simulink model "EHB_MOTOR"  (R2023b)
settings: Solver=FixedStepDiscrete  StartTime=0.0  StopTime=inf  FixedStep=0.0001  RelTol=1e-3  EnableMultiTasking=on
undefined symbols (not defined in the file): CAN_EHB_VCU0x125, CAN_EHB_VCU0x126, CAN_id0x120_Data, Cos_Table, Cos_Table1, EHB_DTC_status, R, Sin_BreakPoint, Sin_BreakPoint1, Sin_Table, Sin_Table1, T
libraries: simulink x30
(part 2 of 9)

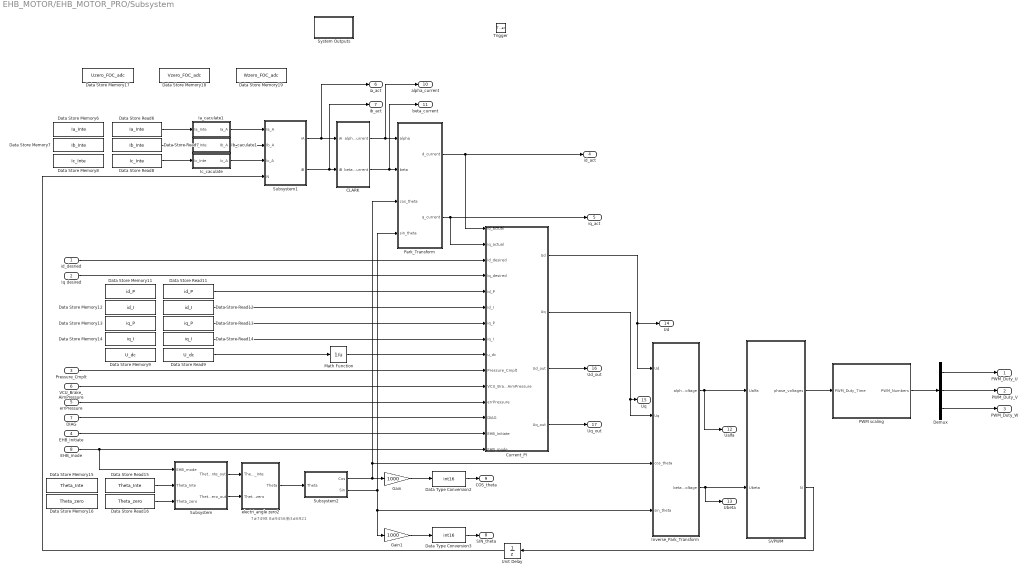
== system EHB_MOTOR/EHB_MOTOR_PRO/Subsystem ==
  note: 7#7498
      | 8#9456
      | 新3#6921
  id_desried : Inport
  Iq desired : Inport  Port=2  OutDataTypeStr=single
  Pressure_Cmplt : Inport  Port=3
  EHB_Initiate : Inport  Port=4
  errPressure : Inport  Port=5
  VCU_Brake_AimPressure : Inport  Port=6
  DIAG : Inport  Port=7
  EHB_mode : Inport  Port=8
  Trigger : TriggerPort  TriggerType=function-call  VariantControl=Variant  PortDimensions=1
  CLARK : Subsystem
  Current_PI : Subsystem
  Data Store Memory11 : DataStoreMemory  DataStoreName=id_P  ReadBeforeWriteMsg=warning  WriteAfterWriteMsg=warning  WriteAfterReadMsg=warning  ShowAdditionalParam=off  OutDataTypeStr=single
  Data Store Memory12 : DataStoreMemory  DataStoreName=id_I  ReadBeforeWriteMsg=warning  WriteAfterWriteMsg=warning  WriteAfterReadMsg=warning  ShowAdditionalParam=off  OutDataTypeStr=single
  Data Store Memory13 : DataStoreMemory  DataStoreName=iq_P  ReadBeforeWriteMsg=warning  WriteAfterWriteMsg=warning  WriteAfterReadMsg=warning  ShowAdditionalParam=off  OutDataTypeStr=single
  Data Store Memory14 : DataStoreMemory  DataStoreName=iq_I  ReadBeforeWriteMsg=warning  WriteAfterWriteMsg=warning  WriteAfterReadMsg=warning  ShowAdditionalParam=off  OutDataTypeStr=single
  Data Store Memory15 : DataStoreMemory  DataStoreName=Theta_Inte  ReadBeforeWriteMsg=warning  WriteAfterWriteMsg=warning  WriteAfterReadMsg=warning  ShowAdditionalParam=off  OutDataTypeStr=uint16
  Data Store Memory16 : DataStoreMemory  DataStoreName=Theta_zero  ReadBeforeWriteMsg=warning  WriteAfterWriteMsg=warning  WriteAfterReadMsg=warning  ShowAdditionalParam=off  OutDataTypeStr=uint16
  Data Store Memory17 : DataStoreMemory  DataStoreName=Uzero_FOC_adc  ReadBeforeWriteMsg=warning  WriteAfterWriteMsg=warning  WriteAfterReadMsg=warning  ShowAdditionalParam=off  OutDataTypeStr=uint16
  Data Store Memory18 : DataStoreMemory  DataStoreName=Vzero_FOC_adc  ReadBeforeWriteMsg=warning  WriteAfterWriteMsg=warning  WriteAfterReadMsg=warning  ShowAdditionalParam=off  OutDataTypeStr=uint16
  Data Store Memory19 : DataStoreMemory  DataStoreName=Wzero_FOC_adc  ReadBeforeWriteMsg=warning  WriteAfterWriteMsg=warning  WriteAfterReadMsg=warning  ShowAdditionalParam=off  OutDataTypeStr=uint16
  Data Store Memory6 : DataStoreMemory  DataStoreName=Ia_Inte  ReadBeforeWriteMsg=warning  WriteAfterWriteMsg=warning  WriteAfterReadMsg=warning  ShowAdditionalParam=off  OutDataTypeStr=uint16
  Data Store Memory7 : DataStoreMemory  DataStoreName=Ib_Inte  ReadBeforeWriteMsg=warning  WriteAfterWriteMsg=warning  WriteAfterReadMsg=warning  ShowAdditionalParam=off  OutDataTypeStr=uint16
  Data Store Memory8 : DataStoreMemory  DataStoreName=Ic_Inte  ReadBeforeWriteMsg=warning  WriteAfterWriteMsg=warning  WriteAfterReadMsg=warning  ShowAdditionalParam=off  OutDataTypeStr=uint16
  Data Store Memory9 : DataStoreMemory  DataStoreName=U_dc  ReadBeforeWriteMsg=warning  WriteAfterWriteMsg=warning  WriteAfterReadMsg=warning  ShowAdditionalParam=off  OutDataTypeStr=single
  Data Store Read11 : DataStoreRead  DataStoreName=id_P  DataStoreElements=id_P  IndexOptions=Index vector (dialog)  Indices=1  OutputSizes=1
  Data Store Read12 : DataStoreRead  DataStoreName=id_I  DataStoreElements=id_I  IndexOptions=Index vector (dialog)  Indices=1  OutputSizes=1
  Data Store Read13 : DataStoreRead  DataStoreName=iq_P  DataStoreElements=iq_P  IndexOptions=Index vector (dialog)  Indices=1  OutputSizes=1
  Data Store Read14 : DataStoreRead  DataStoreName=iq_I  DataStoreElements=iq_I  IndexOptions=Index vector (dialog)  Indices=1  OutputSizes=1
  Data Store Read15 : DataStoreRead  DataStoreName=Theta_Inte  DataStoreElements=Theta_Inte  IndexOptions=Index vector (dialog)  Indices=1  OutputSizes=1
  Data Store Read16 : DataStoreRead  DataStoreName=Theta_zero  DataStoreElements=Theta_zero  IndexOptions=Index vector (dialog)  Indices=1  OutputSizes=1
  Data Store Read6 : DataStoreRead  DataStoreName=Ia_Inte  DataStoreElements=Ia_Inte  IndexOptions=Index vector (dialog)  Indices=1  OutputSizes=1
  Data Store Read7 : DataStoreRead  DataStoreName=Ib_Inte  DataStoreElements=Ib_Inte  IndexOptions=Index vector (dialog)  Indices=1  OutputSizes=1
  Data Store Read8 : DataStoreRead  DataStoreName=Ic_Inte  DataStoreElements=Ic_Inte  IndexOptions=Index vector (dialog)  Indices=1  OutputSizes=1
  Data Store Read9 : DataStoreRead  DataStoreName=U_dc  DataStoreElements=U_dc  IndexOptions=Index vector (dialog)  Indices=1  OutputSizes=1
  Data Type Conversion2 : DataTypeConversion  OutDataTypeStr=int16  SaturateOnIntegerOverflow=off  RndMeth=Floor
  Data Type Conversion3 : DataTypeConversion  OutDataTypeStr=int16  SaturateOnIntegerOverflow=off  RndMeth=Floor
  Demux : Demux  Outputs=3
  Gain : Gain  Gain=1000
  Gain1 : Gain  Gain=1000
  Ia_caculate1 : Subsystem
  Ib_caculate1 : Subsystem
  Ic_caculate : Subsystem
  Inverse_Park_Transform : Subsystem
  Math Function : Math  Operator=reciprocal  SignedPower=on  OutDataTypeStr=single
  PWM scaling : Subsystem
  Park_Transform : Subsystem
  SVPWM : Subsystem
  Subsystem : Subsystem
  Subsystem1 : Subsystem
  Subsystem2 : Subsystem
  System Outputs : Subsystem  mask(System Outputs){ShowInLibBrowser=0}
      mask prompts: ShowInLibBrowser "Simulink:masks:CustCodeMaskParam1_MP"
      settings: CopyFcn=cccopyfcn(gcb)  OpenFcn=ccopenfcn('System Outputs Function')
      mask Help: eval('feval(''rtwprivate'',''rtwhelpview'',''rtw_sys_outputs_block'')');
      mask Display: disp('System\nOutputs');
  Unit Delay : UnitDelay  SampleTime=-1  HasFrameUpgradeWarning=on
  electri_angle zero2 : Subsystem
  PWM_Duty_U : Outport  VectorParamsAs1DForOutWhenUnconnected=off
  PWM_Duty_V : Outport  Port=2  VectorParamsAs1DForOutWhenUnconnected=off
  PWM_Duty_W : Outport  Port=3  VectorParamsAs1DForOutWhenUnconnected=off
  id_act : Outport  Port=4  VectorParamsAs1DForOutWhenUnconnected=off
  iq_act : Outport  Port=5  VectorParamsAs1DForOutWhenUnconnected=off
  ia_act : Outport  Port=6  OutDataTypeStr=single  VectorParamsAs1DForOutWhenUnconnected=off
  ib_act : Outport  Port=7  OutDataTypeStr=single  VectorParamsAs1DForOutWhenUnconnected=off
  SIN_theta : Outport  Port=8  VectorParamsAs1DForOutWhenUnconnected=off
  COS_theta : Outport  Port=9  VectorParamsAs1DForOutWhenUnconnected=off
  alpha_current : Outport  Port=10  OutDataTypeStr=single  VectorParamsAs1DForOutWhenUnconnected=off
  beta_current : Outport  Port=11  OutDataTypeStr=single  VectorParamsAs1DForOutWhenUnconnected=off
  Ualfa : Outport  Port=12  VectorParamsAs1DForOutWhenUnconnected=off
  Ubeta : Outport  Port=13  VectorParamsAs1DForOutWhenUnconnected=off
  Ud : Outport  Port=14  VectorParamsAs1DForOutWhenUnconnected=off
  Uq : Outport  Port=15  VectorParamsAs1DForOutWhenUnconnected=off
  Ud_out : Outport  Port=16  OutDataTypeStr=single  VectorParamsAs1DForOutWhenUnconnected=off
  Uq_out : Outport  Port=17  OutDataTypeStr=single  VectorParamsAs1DForOutWhenUnconnected=off
  wires:
  Inverse_Park_Transform/2(beta_voltage) -> Ubeta/1, SVPWM/2(Ubeta)
  Iq desired/1 -> Current_PI/4(Iq_desired)
  Data Store Read13/1 -> Current_PI/7(iq_P)
  CLARK/1(alpha_current) -> alpha_current/1, Park_Transform/1(alpha)
  Demux/1 -> PWM_Duty_U/1
  CLARK/2(beta_current) -> beta_current/1, Park_Transform/2(beta)
  Data Store Read12/1 -> Current_PI/6(id_I)
  Data Store Read14/1 -> Current_PI/8(iq_I)
  Park_Transform/2(q_current) -> Current_PI/2(iq_actual), iq_act/1
  Current_PI/2(Uq) -> Inverse_Park_Transform/2(Uq), Uq/1
  Data Store Read11/1 -> Current_PI/5(id_P)
  Math Function/1 -> Current_PI/9(u_dc)
  Gain1/1 -> Data Type Conversion3/1
  Gain/1 -> Data Type Conversion2/1
  Inverse_Park_Transform/1(alpha_voltage) -> Ualfa/1, SVPWM/1(Ualfa)
  Current_PI/1(Ud) -> Inverse_Park_Transform/1(Ud), Ud/1
  Data Type Conversion3/1 -> SIN_theta/1
  Subsystem1/1(iA) -> ia_act/1, CLARK/1(iA)
  PWM scaling/1(PWM_Numbers) -> Demux/1
  Park_Transform/1(d_current) -> Current_PI/1(id_actual), id_act/1
  Subsystem1/2(iB) -> ib_act/1, CLARK/2(iB)
  Demux/3 -> PWM_Duty_W/1
  Data Store Read7/1 -> Ib_caculate1/1(Ib_Inte)
  Data Store Read6/1 -> Ia_caculate1/1(Ia_Inte)
  Data Store Read9/1 -> Math Function/1
  Demux/2 -> PWM_Duty_V/1
  Data Type Conversion2/1 -> COS_theta/1
  id_desried/1 -> Current_PI/3(id_desired)
  SVPWM/1(phase_voltages) -> PWM scaling/1(PWM_Duty_Time)
  Pressure_Cmplt/1 -> Current_PI/10(Pressure_Cmplt)
  VCU_Brake_AimPressure/1 -> Current_PI/11(VCU_Brake_AimPressure)
  Ib_caculate1/1(Ib_A) -> Subsystem1/2(Ib_A)
  Ia_caculate1/1(Ia_A) -> Subsystem1/1(Ia_A)
  Ic_caculate/1(Ic_A) -> Subsystem1/3(Ic_A)
  Data Store Read8/1 -> Ic_caculate/1(Ic_Inte)
  SVPWM/2(N) -> Unit Delay/1
  Unit Delay/1 -> Subsystem1/4(N)
  Subsystem2/1(Cos) -> Park_Transform/3(cos_theta), Inverse_Park_Transform/3(cos_theta), Gain/1
  Subsystem2/2(Sin) -> Gain1/1, Inverse_Park_Transform/4(sin_theta), Park_Transform/4(sin_theta)
  electri_angle zero2/1(Theta) -> Subsystem2/1(Theta)
  errPressure/1 -> Current_PI/12(errPressure)
  DIAG/1 -> Current_PI/13(DIAG)
  EHB_Initiate/1 -> Current_PI/14(EHB_Initiate)
  EHB_mode/1 -> Subsystem/1(EHB_mode), Current_PI/15(EHB_mode)
  Data Store Read15/1 -> Subsystem/2(Theta_Inte)
  Data Store Read16/1 -> Subsystem/3(Theta_zero)
  Subsystem/1(Theta_Inte_out) -> electri_angle zero2/1(Theta_Inte)
  Subsystem/2(Theta_zero_out) -> electri_angle zero2/2(Theta_zero)
  Current_PI/4(Uq_out) -> Uq_out/1
  Current_PI/3(Ud_out) -> Ud_out/1

== system EHB_MOTOR/EPB_CTRL/EPB_CTRL ==
  EPB_CMD : Inport
  EPB_DiagBUS : Inport  Port=2
  EPB_INPUTBUS : Inport  Port=3
  Trigger : TriggerPort  TriggerType=function-call  VariantControl=Variant  PortDimensions=1
  Bus Selector : BusSelector  OutputSignals=EPB1_Current_filtered,EPB2_Current_filtered
  Chart : Stateflow chart  TreatAsAtomicUnit=on
  Constant : Constant  Value=0  OutDataTypeStr=uint8
  Data Store Memory1 : DataStoreMemory  DataStoreName=EPB_tiRelease_C  ReadBeforeWriteMsg=warning  WriteAfterWriteMsg=warning  WriteAfterReadMsg=warning  ShowAdditionalParam=off  OutDataTypeStr=uint16
  Data Store Memory2 : DataStoreMemory  DataStoreName=EPB_tiClamp_C  ReadBeforeWriteMsg=warning  WriteAfterWriteMsg=warning  WriteAfterReadMsg=warning  ShowAdditionalParam=off  OutDataTypeStr=uint16
  Data Store Memory3 : DataStoreMemory  DataStoreName=EPB1_iAct_C  ReadBeforeWriteMsg=warning  WriteAfterWriteMsg=warning  WriteAfterReadMsg=warning  ShowAdditionalParam=off  OutDataTypeStr=single
  Data Store Memory4 : DataStoreMemory  DataStoreName=EPB2_iAct_C  ReadBeforeWriteMsg=warning  WriteAfterWriteMsg=warning  WriteAfterReadMsg=warning  ShowAdditionalParam=off  OutDataTypeStr=single
  Data Store Read : DataStoreRead  DataStoreName=EPB_tiClamp_C  DataStoreElements=EPB_tiClamp_C  IndexOptions=Index vector (dialog)  Indices=1  OutputSizes=1
  Data Store Read1 : DataStoreRead  DataStoreName=EPB_tiRelease_C  DataStoreElements=EPB_tiRelease_C  IndexOptions=Index vector (dialog)  Indices=1  OutputSizes=1
  Data Store Read2 : DataStoreRead  DataStoreName=EPB1_iAct_C  DataStoreElements=EPB1_iAct_C  IndexOptions=Index vector (dialog)  Indices=1  OutputSizes=1
  Data Store Read3 : DataStoreRead  DataStoreName=EPB2_iAct_C  DataStoreElements=EPB2_iAct_C  IndexOptions=Index vector (dialog)  Indices=1  OutputSizes=1
  Fault_Handle : Subsystem
  Switch : Switch  Criteria=u2 ~= 0  SaturateOnIntegerOverflow=off  InputSameDT=off
  EPB_PWMout : Outport  VectorParamsAs1DForOutWhenUnconnected=off
  EPB_state : Outport  Port=2  VectorParamsAs1DForOutWhenUnconnected=off
  Clamp_ok : Outport  Port=3  VectorParamsAs1DForOutWhenUnconnected=off
  Release_ok : Outport  Port=4  VectorParamsAs1DForOutWhenUnconnected=off
  wires:
  EPB_INPUTBUS/1 -> Bus Selector/1
  EPB_CMD/1 -> Chart/1(EPB_Ctrl_Req)
  Bus Selector/1 -> Chart/2(EPB1_iAct)  "<EPB1_Current_filtered>"
  Bus Selector/2 -> Chart/3(EPB2_iAct)  "<EPB2_Current_filtered>"
  Data Store Read/1 -> Chart/4(EPB_tiClamp_C)
  Data Store Read1/1 -> Chart/5(EPB_tiRelease_C)
  Data Store Read2/1 -> Chart/6(EPB1_iAct_C)
  Data Store Read3/1 -> Chart/7(EPB2_iAct_C)
  Chart/1(EPB_PWMout) -> Switch/3
  Chart/2(EPB_dir_state) -> EPB_state/1
  Chart/3(Clamp_ok) -> Clamp_ok/1
  Chart/4(Release_ok) -> Release_ok/1
  EPB_DiagBUS/1 -> Fault_Handle/1(In1)
  Fault_Handle/1(Out1) -> Switch/2
  Constant/1 -> Switch/1
  Switch/1 -> EPB_PWMout/1

== system EHB_MOTOR/EPB_CTRL/EPB_Diag ==
  In1 : Inport
  Trigger : TriggerPort  TriggerType=function-call  VariantControl=Variant  PortDimensions=1
  Bus Creator : BusCreator  Inputs=4
  Bus Selector13 : BusSelector  OutputSignals=EPB1_Current_filtered,EPB2_Current_filtered
  Bus Selector15 : BusSelector  OutputSignals=EPB1_Temp
  Bus Selector5 : BusSelector  OutputSignals=EPB_vBAT_filtered
  EPBCurrentDiag : Subsystem
  EPBOverheatDiag : Subsystem
  EPB_vBATDiag : Subsystem
  EPB_DiagBUS : Outport  VectorParamsAs1DForOutWhenUnconnected=off
  wires:
  Bus Selector5/1 -> EPB_vBATDiag/1(EPBVoltage)  "<EPB_vBAT_filtered>"
  Bus Selector15/1 -> EPBOverheatDiag/1(EPBTemp)  "<EPB1_Temp>"
  Bus Selector13/2 -> EPBCurrentDiag/2(EPB2Current)  "<EPB2_Current_filtered>"
  Bus Selector13/1 -> EPBCurrentDiag/1(EPB1Current)  "<EPB1_Current_filtered>"
  In1/1 -> Bus Selector13/1, Bus Selector15/1, Bus Selector5/1
  EPB_vBATDiag/1(EPBVoltageLow) -> Bus Creator/1  "EPBVoltageLow"
  EPB_vBATDiag/2(EPBVoltageHigh) -> Bus Creator/2  "EPBVoltageHigh"
  EPBOverheatDiag/1(EPBOverheat) -> Bus Creator/3  "EPBOverheat"
  EPBCurrentDiag/1(EPBCurrentOverride) -> Bus Creator/4  "EPBCurrentOverride"
  Bus Creator/1 -> EPB_DiagBUS/1

== system EHB_MOTOR/EPB_CTRL/Subsystem1 ==
  Trigger : TriggerPort  TriggerType=function-call  VariantControl=Variant  PortDimensions=1
  Bus Creator : BusCreator  Inputs=11
  Data Store Memory11 : DataStoreMemory  DataStoreName=EPB_vBAT_AD  ReadBeforeWriteMsg=warning  WriteAfterWriteMsg=warning  WriteAfterReadMsg=warning  ShowAdditionalParam=off  OutDataTypeStr=uint16
  Data Store Memory12 : DataStoreMemory  DataStoreName=EPB1_Temp_AD  ReadBeforeWriteMsg=warning  WriteAfterWriteMsg=warning  WriteAfterReadMsg=warning  ShowAdditionalParam=off  OutDataTypeStr=uint16
  Data Store Memory13 : DataStoreMemory  DataStoreName=EPB_APBSwitch2_AD  ReadBeforeWriteMsg=warning  WriteAfterWriteMsg=warning  WriteAfterReadMsg=warning  ShowAdditionalParam=off  OutDataTypeStr=uint16
  Data Store Memory14 : DataStoreMemory  DataStoreName=EPB_7181PreDriver1_AD  ReadBeforeWriteMsg=warning  WriteAfterWriteMsg=warning  WriteAfterReadMsg=warning  ShowAdditionalParam=off  OutDataTypeStr=uint16
  Data Store Memory15 : DataStoreMemory  DataStoreName=EPB2_Temp_AD  ReadBeforeWriteMsg=warning  WriteAfterWriteMsg=warning  WriteAfterReadMsg=warning  ShowAdditionalParam=off  OutDataTypeStr=uint16
  Data Store Memory17 : DataStoreMemory  DataStoreName=EPB_APBSwitch3_AD  ReadBeforeWriteMsg=warning  WriteAfterWriteMsg=warning  WriteAfterReadMsg=warning  ShowAdditionalParam=off  OutDataTypeStr=uint16
  Data Store Memory18 : DataStoreMemory  DataStoreName=EPB_APBSwitch4_AD  ReadBeforeWriteMsg=warning  WriteAfterWriteMsg=warning  WriteAfterReadMsg=warning  ShowAdditionalParam=off  OutDataTypeStr=uint16
  Data Store Memory19 : DataStoreMemory  DataStoreName=EPB2_Current_AD  ReadBeforeWriteMsg=warning  WriteAfterWriteMsg=warning  WriteAfterReadMsg=warning  ShowAdditionalParam=off  OutDataTypeStr=uint16
  Data Store Memory20 : DataStoreMemory  DataStoreName=EPB_APBSwitch1_AD  ReadBeforeWriteMsg=warning  WriteAfterWriteMsg=warning  WriteAfterReadMsg=warning  ShowAdditionalParam=off  OutDataTypeStr=uint16
  Data Store Memory21 : DataStoreMemory  DataStoreName=EPB1_Current_AD  ReadBeforeWriteMsg=warning  WriteAfterWriteMsg=warning  WriteAfterReadMsg=warning  ShowAdditionalParam=off  OutDataTypeStr=uint16
  Data Store Memory22 : DataStoreMemory  DataStoreName=EPB_7181PreDriver2_AD  ReadBeforeWriteMsg=warning  WriteAfterWriteMsg=warning  WriteAfterReadMsg=warning  ShowAdditionalParam=off  OutDataTypeStr=uint16
  Data Store Read11 : DataStoreRead  DataStoreName=EPB_vBAT_AD  DataStoreElements=EPB_vBAT_AD  IndexOptions=Index vector (dialog)  Indices=1  OutputSizes=1
  Data Store Read12 : DataStoreRead  DataStoreName=EPB1_Temp_AD  DataStoreElements=EPB1_Temp_AD  IndexOptions=Index vector (dialog)  Indices=1  OutputSizes=1
  Data Store Read13 : DataStoreRead  DataStoreName=EPB_APBSwitch2_AD  DataStoreElements=EPB_APBSwitch2_AD  IndexOptions=Index vector (dialog)  Indices=1  OutputSizes=1
  Data Store Read14 : DataStoreRead  DataStoreName=EPB_7181PreDriver1_AD  DataStoreElements=EPB_7181PreDriver1_AD  IndexOptions=Index vector (dialog)  Indices=1  OutputSizes=1
  Data Store Read15 : DataStoreRead  DataStoreName=EPB2_Temp_AD  DataStoreElements=EPB2_Temp_AD  IndexOptions=Index vector (dialog)  Indices=1  OutputSizes=1
  Data Store Read17 : DataStoreRead  DataStoreName=EPB_APBSwitch3_AD  DataStoreElements=EPB_APBSwitch3_AD  IndexOptions=Index vector (dialog)  Indices=1  OutputSizes=1
  Data Store Read18 : DataStoreRead  DataStoreName=EPB_APBSwitch4_AD  DataStoreElements=EPB_APBSwitch4_AD  IndexOptions=Index vector (dialog)  Indices=1  OutputSizes=1
  Data Store Read19 : DataStoreRead  DataStoreName=EPB2_Current_AD  DataStoreElements=EPB2_Current_AD  IndexOptions=Index vector (dialog)  Indices=1  OutputSizes=1
  Data Store Read20 : DataStoreRead  DataStoreName=EPB_APBSwitch1_AD  DataStoreElements=EPB_APBSwitch1_AD  IndexOptions=Index vector (dialog)  Indices=1  OutputSizes=1
  Data Store Read21 : DataStoreRead  DataStoreName=EPB1_Current_AD  DataStoreElements=EPB1_Current_AD  IndexOptions=Index vector (dialog)  Indices=1  OutputSizes=1
  Data Store Read22 : DataStoreRead  DataStoreName=EPB_7181PreDriver2_AD  DataStoreElements=EPB_7181PreDriver2_AD  IndexOptions=Index vector (dialog)  Indices=1  OutputSizes=1
  EPB_interface : Subsystem
  EPB_INPUTBUS : Outport  VectorParamsAs1DForOutWhenUnconnected=off
  wires:
  Data Store Read21/1 -> EPB_interface/2(EPB1_Current_AD)
  Data Store Read17/1 -> EPB_interface/6(EPB_APBSwitch3_AD)
  Data Store Read14/1 -> EPB_interface/11(EPB_7181PreDriver1_AD)
  Data Store Read13/1 -> EPB_interface/10(EPB_7181PreDriver2_AD)
  EPB_interface/9(EPB_APBSwitch2_filtered) -> Bus Creator/9  "EPB_7181PreDriver2_filtered"
  Data Store Read19/1 -> EPB_interface/3(EPB2_Current_AD)
  Data Store Read12/1 -> EPB_interface/4(EPB1_Temp_AD)
  Data Store Read22/1 -> EPB_interface/9(EPB_APBSwitch2_AD)
  Data Store Read15/1 -> EPB_interface/5(EPB2_Temp_AD)
  Data Store Read20/1 -> EPB_interface/8(EPB_APBSwitch1_AD)
  EPB_interface/7(EPB_APBSwitch4_filtered) -> Bus Creator/7  "EPB_APBSwitch4_filtered"
  EPB_interface/11(EPB_7181PreDriver1_filtered) -> Bus Creator/11  "EPB_7181PreDriver1_filtered"
  EPB_interface/4(EPB1_Temp) -> Bus Creator/4  "EPB1_Temp"
  EPB_interface/3(EPB2_Current_filtered) -> Bus Creator/3  "EPB2_Current_filtered"
  Data Store Read11/1 -> EPB_interface/1(EPB_vBAT_AD)
  EPB_interface/2(EPB1_Current_filtered) -> Bus Creator/2  "EPB1_Current_filtered"
  Data Store Read18/1 -> EPB_interface/7(EPB_APBSwitch4_AD)
  EPB_interface/6(EPB_APBSwitch3_filtered) -> Bus Creator/6  "EPB_APBSwitch3_filtered"
  EPB_interface/5(EPB2_Temp) -> Bus Creator/5  "EPB2_Temp"
  EPB_interface/1(EPB_vBAT_filtered) -> Bus Creator/1  "EPB_vBAT_filtered"
  EPB_interface/10(EPB_7181PreDriver2_filtered) -> Bus Creator/10  "EPB_APBSwitch2_filtered"
  EPB_interface/8(EPB_APBSwitch1_filtered) -> Bus Creator/8  "EPB_APBSwitch1_filtered"
  Bus Creator/1 -> EPB_INPUTBUS/1

== system EHB_MOTOR/EHB_MOTOR_PRO/DIAG/5vDiag ==
  note: 20ms
  note: 5v输出异常
  5vVoltage : Inport
  Chart : Stateflow chart  TreatAsAtomicUnit=on
  Subsystem : Subsystem
  5vErr : Outport  VectorParamsAs1DForOutWhenUnconnected=off
  wires:
  5vVoltage/1 -> Subsystem/1(In1)
  Subsystem/1(Out1) -> 5vErr/1
  Chart/1(task_20ms()) -> Subsystem/Trigger

== system EHB_MOTOR/EHB_MOTOR_PRO/DIAG/AngleSensorDiag ==
  note: 角度传感器缺少标定
  note: 角度传感器没有信号
  note: 200ms
  note: 角度传感器信号超限故障
  note: 200ms
  note: 200ms
  AngleSensorSignal : Inport
  AngleSensorCalFlag : Inport  Port=2
  Chart : Stateflow chart  TreatAsAtomicUnit=on
  Chart1 : Stateflow chart  TreatAsAtomicUnit=on
  Chart2 : Stateflow chart  TreatAsAtomicUnit=on
  Subsystem : Subsystem
  Subsystem1 : Subsystem
  Subsystem2 : Subsystem
  AngleSensorSignalOverride : Outport  VectorParamsAs1DForOutWhenUnconnected=off
  AngleSensorSignalLost : Outport  Port=2  VectorParamsAs1DForOutWhenUnconnected=off
  AngleSensorNoCal : Outport  Port=3  VectorParamsAs1DForOutWhenUnconnected=off
  wires:
  Subsystem/1(Out1) -> AngleSensorSignalOverride/1
  Chart/1(task_200ms()) -> Subsystem/Trigger
  Chart1/1(task_200ms()) -> Subsystem1/Trigger
  Subsystem1/1(Out1) -> AngleSensorSignalLost/1
  AngleSensorSignal/1 -> Subsystem1/1(In1), Subsystem/1(In1)
  Subsystem2/1(Out1) -> AngleSensorNoCal/1
  Chart2/1(task_200ms()) -> Subsystem2/Trigger
  AngleSensorCalFlag/1 -> Subsystem2/1(In1)

== system EHB_MOTOR/EHB_MOTOR_PRO/DIAG/BusOffDiag ==
  note: 控制器内部故障
  In1 : Inport
  Ground : Ground
  Terminator : Terminator
  BusOffErr : Outport  VectorParamsAs1DForOutWhenUnconnected=off
  wires:
  In1/1 -> Terminator/1
  Ground/1 -> BusOffErr/1

== system EHB_MOTOR/EHB_MOTOR_PRO/DIAG/CANCommDiag ==
  note: CAN收发模块故障
  In1 : Inport
  Ground : Ground
  Terminator : Terminator
  CANCommErr : Outport  VectorParamsAs1DForOutWhenUnconnected=off
  wires:
  In1/1 -> Terminator/1
  Ground/1 -> CANCommErr/1

== system EHB_MOTOR/EHB_MOTOR_PRO/DIAG/CANDataLostDiag ==
  note: CAN丢失数据
  In1 : Inport
  Ground : Ground
  Terminator : Terminator
  CANDataLostErr : Outport  VectorParamsAs1DForOutWhenUnconnected=off
  wires:
  In1/1 -> Terminator/1
  Ground/1 -> CANDataLostErr/1

== system EHB_MOTOR/EHB_MOTOR_PRO/DIAG/Chip7189Diag ==
  note: 7189芯片故障
  note: 20ms
  Chart : Stateflow chart  TreatAsAtomicUnit=on
  Data Store Memory1 : DataStoreMemory  DataStoreName=Chip7189ErrFlag  ReadBeforeWriteMsg=warning  WriteAfterWriteMsg=warning  WriteAfterReadMsg=warning  ShowAdditionalParam=off  OutDataTypeStr=uint8
  Data Store Read2 : DataStoreRead  DataStoreName=Chip7189ErrFlag  DataStoreElements=Chip7189ErrFlag  IndexOptions=Index vector (dialog)  Indices=1  OutputSizes=1
  Subsystem : Subsystem
  Chip7189_err : Outport  VectorParamsAs1DForOutWhenUnconnected=off
  wires:
  Chart/1(task_20ms()) -> Subsystem/Trigger
  Subsystem/1(Out1) -> Chip7189_err/1
  Data Store Read2/1 -> Subsystem/1(In1)

== system EHB_MOTOR/EHB_MOTOR_PRO/DIAG/CurrentSensorDiag ==
  note: 200ms
  note: U相电流传感器故障
  note: 200ms
  note: V相电流传感器故障
  note: 200ms
  note: W相电流传感器故障
  CurrentSensorU : Inport
  CurrentSensorV : Inport  Port=2
  CurrentSensorW : Inport  Port=3
  Chart : Stateflow chart  TreatAsAtomicUnit=on
  Chart1 : Stateflow chart  TreatAsAtomicUnit=on
  Chart2 : Stateflow chart  TreatAsAtomicUnit=on
  Subsystem : Subsystem
  Subsystem1 : Subsystem
  Subsystem2 : Subsystem
  CurrentSensorUOverride : Outport  VectorParamsAs1DForOutWhenUnconnected=off
  CurrentSensorVOverride : Outport  Port=2  VectorParamsAs1DForOutWhenUnconnected=off
  CurrentSensorWOverride : Outport  Port=3  VectorParamsAs1DForOutWhenUnconnected=off
  wires:
  CurrentSensorU/1 -> Subsystem/1(In1)
  Subsystem/1(Out1) -> CurrentSensorUOverride/1
  Chart/1(task_200ms()) -> Subsystem/Trigger
  Chart1/1(task_200ms()) -> Subsystem1/Trigger
  Subsystem1/1(Out1) -> CurrentSensorVOverride/1
  CurrentSensorV/1 -> Subsystem1/1(In1)
  CurrentSensorW/1 -> Subsystem2/1(In1)
  Subsystem2/1(Out1) -> CurrentSensorWOverride/1
  Chart2/1(task_200ms()) -> Subsystem2/Trigger

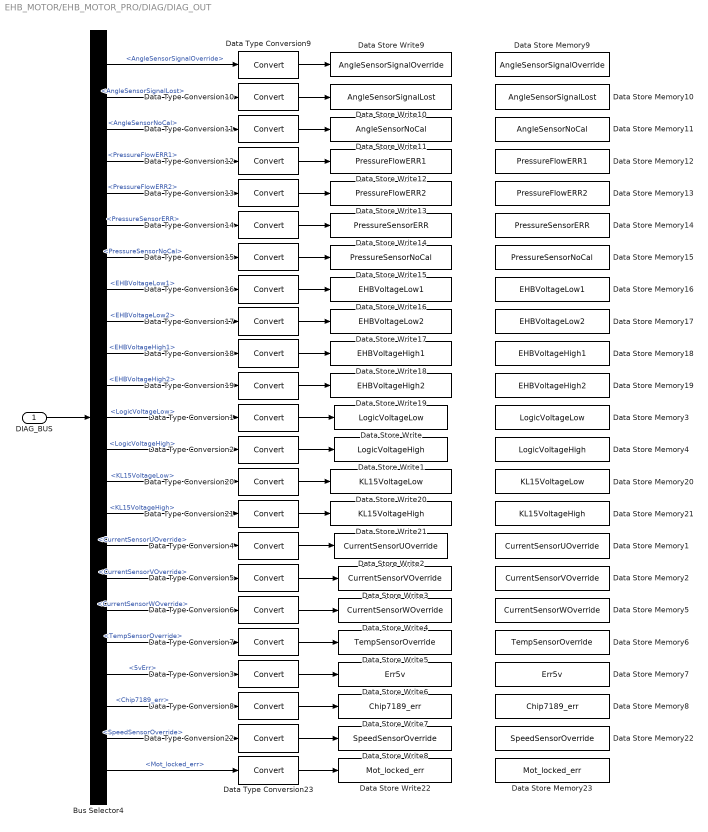
== system EHB_MOTOR/EHB_MOTOR_PRO/DIAG/DIAG_OUT ==
  DIAG_BUS : Inport
  Bus Selector4 : BusSelector  OutputSignals=AngleSensorSignalOverride,AngleSensorSignalLost,AngleSensorNoCal,PressureFlowERR1,PressureFlowERR2,PressureSensorERR,PressureSensorNoCal,EHBVoltageLow1,EHBVoltageLow2,EHBVoltageHigh1,EHBVoltageHigh2,LogicVoltageLow,LogicVoltageHigh,KL15VoltageLow,KL15VoltageHigh,CurrentSensorUOverride,CurrentSensorVOverride,CurrentSensorWOverride,TempSensorOverride,5vErr,Chip7189_err,SpeedSensorOverride,Mot_locked_err
  Data Store Memory1 : DataStoreMemory  DataStoreName=CurrentSensorUOverride  ReadBeforeWriteMsg=warning  WriteAfterWriteMsg=warning  WriteAfterReadMsg=warning  ShowAdditionalParam=off  OutDataTypeStr=uint8
  Data Store Memory10 : DataStoreMemory  DataStoreName=AngleSensorSignalLost  ReadBeforeWriteMsg=warning  WriteAfterWriteMsg=warning  WriteAfterReadMsg=warning  ShowAdditionalParam=off  OutDataTypeStr=uint8
  Data Store Memory11 : DataStoreMemory  DataStoreName=AngleSensorNoCal  ReadBeforeWriteMsg=warning  WriteAfterWriteMsg=warning  WriteAfterReadMsg=warning  ShowAdditionalParam=off  OutDataTypeStr=uint8
  Data Store Memory12 : DataStoreMemory  DataStoreName=PressureFlowERR1  ReadBeforeWriteMsg=warning  WriteAfterWriteMsg=warning  WriteAfterReadMsg=warning  ShowAdditionalParam=off  OutDataTypeStr=uint8
  Data Store Memory13 : DataStoreMemory  DataStoreName=PressureFlowERR2  ReadBeforeWriteMsg=warning  WriteAfterWriteMsg=warning  WriteAfterReadMsg=warning  ShowAdditionalParam=off  OutDataTypeStr=uint8
  Data Store Memory14 : DataStoreMemory  DataStoreName=PressureSensorERR  ReadBeforeWriteMsg=warning  WriteAfterWriteMsg=warning  WriteAfterReadMsg=warning  ShowAdditionalParam=off  OutDataTypeStr=uint8
  Data Store Memory15 : DataStoreMemory  DataStoreName=PressureSensorNoCal  ReadBeforeWriteMsg=warning  WriteAfterWriteMsg=warning  WriteAfterReadMsg=warning  ShowAdditionalParam=off  OutDataTypeStr=uint8
  Data Store Memory16 : DataStoreMemory  DataStoreName=EHBVoltageLow1  ReadBeforeWriteMsg=warning  WriteAfterWriteMsg=warning  WriteAfterReadMsg=warning  ShowAdditionalParam=off  OutDataTypeStr=uint8
  Data Store Memory17 : DataStoreMemory  DataStoreName=EHBVoltageLow2  ReadBeforeWriteMsg=warning  WriteAfterWriteMsg=warning  WriteAfterReadMsg=warning  ShowAdditionalParam=off  OutDataTypeStr=uint8
  Data Store Memory18 : DataStoreMemory  DataStoreName=EHBVoltageHigh1  ReadBeforeWriteMsg=warning  WriteAfterWriteMsg=warning  WriteAfterReadMsg=warning  ShowAdditionalParam=off  OutDataTypeStr=uint8
  Data Store Memory19 : DataStoreMemory  DataStoreName=EHBVoltageHigh2  ReadBeforeWriteMsg=warning  WriteAfterWriteMsg=warning  WriteAfterReadMsg=warning  ShowAdditionalParam=off  OutDataTypeStr=uint8
  Data Store Memory2 : DataStoreMemory  DataStoreName=CurrentSensorVOverride  ReadBeforeWriteMsg=warning  WriteAfterWriteMsg=warning  WriteAfterReadMsg=warning  ShowAdditionalParam=off  OutDataTypeStr=uint8
  Data Store Memory20 : DataStoreMemory  DataStoreName=KL15VoltageLow  ReadBeforeWriteMsg=warning  WriteAfterWriteMsg=warning  WriteAfterReadMsg=warning  ShowAdditionalParam=off  OutDataTypeStr=uint8
  Data Store Memory21 : DataStoreMemory  DataStoreName=KL15VoltageHigh  ReadBeforeWriteMsg=warning  WriteAfterWriteMsg=warning  WriteAfterReadMsg=warning  ShowAdditionalParam=off  OutDataTypeStr=uint8
  Data Store Memory22 : DataStoreMemory  DataStoreName=SpeedSensorOverride  ReadBeforeWriteMsg=warning  WriteAfterWriteMsg=warning  WriteAfterReadMsg=warning  ShowAdditionalParam=off  OutDataTypeStr=uint8
  Data Store Memory23 : DataStoreMemory  DataStoreName=Mot_locked_err  ReadBeforeWriteMsg=warning  WriteAfterWriteMsg=warning  WriteAfterReadMsg=warning  ShowAdditionalParam=off  OutDataTypeStr=uint8
  Data Store Memory3 : DataStoreMemory  DataStoreName=LogicVoltageLow  ReadBeforeWriteMsg=warning  WriteAfterWriteMsg=warning  WriteAfterReadMsg=warning  ShowAdditionalParam=off  OutDataTypeStr=uint8
  Data Store Memory4 : DataStoreMemory  DataStoreName=LogicVoltageHigh  ReadBeforeWriteMsg=warning  WriteAfterWriteMsg=warning  WriteAfterReadMsg=warning  ShowAdditionalParam=off  OutDataTypeStr=uint8
  Data Store Memory5 : DataStoreMemory  DataStoreName=CurrentSensorWOverride  ReadBeforeWriteMsg=warning  WriteAfterWriteMsg=warning  WriteAfterReadMsg=warning  ShowAdditionalParam=off  OutDataTypeStr=uint8
  Data Store Memory6 : DataStoreMemory  DataStoreName=TempSensorOverride  ReadBeforeWriteMsg=warning  WriteAfterWriteMsg=warning  WriteAfterReadMsg=warning  ShowAdditionalParam=off  OutDataTypeStr=uint8
  Data Store Memory7 : DataStoreMemory  DataStoreName=Err5v  ReadBeforeWriteMsg=warning  WriteAfterWriteMsg=warning  WriteAfterReadMsg=warning  ShowAdditionalParam=off  OutDataTypeStr=uint8
  Data Store Memory8 : DataStoreMemory  DataStoreName=Chip7189_err  ReadBeforeWriteMsg=warning  WriteAfterWriteMsg=warning  WriteAfterReadMsg=warning  ShowAdditionalParam=off  OutDataTypeStr=uint8
  Data Store Memory9 : DataStoreMemory  DataStoreName=AngleSensorSignalOverride  ReadBeforeWriteMsg=warning  WriteAfterWriteMsg=warning  WriteAfterReadMsg=warning  ShowAdditionalParam=off  OutDataTypeStr=uint8
  Data Store Write : DataStoreWrite  DataStoreName=LogicVoltageLow  IndexOptions=Index vector (dialog)  Indices=1  OutputSizes=1
  Data Store Write1 : DataStoreWrite  DataStoreName=LogicVoltageHigh  IndexOptions=Index vector (dialog)  Indices=1  OutputSizes=1
  Data Store Write10 : DataStoreWrite  DataStoreName=AngleSensorSignalLost  DataStoreElements=AngleSensorSignalLost  IndexOptions=Index vector (dialog)  Indices=1  OutputSizes=1
  Data Store Write11 : DataStoreWrite  DataStoreName=AngleSensorNoCal  DataStoreElements=AngleSensorNoCal  IndexOptions=Index vector (dialog)  Indices=1  OutputSizes=1
  Data Store Write12 : DataStoreWrite  DataStoreName=PressureFlowERR1  DataStoreElements=PressureFlowERR1  IndexOptions=Index vector (dialog)  Indices=1  OutputSizes=1
  Data Store Write13 : DataStoreWrite  DataStoreName=PressureFlowERR2  DataStoreElements=PressureFlowERR2  IndexOptions=Index vector (dialog)  Indices=1  OutputSizes=1
  Data Store Write14 : DataStoreWrite  DataStoreName=PressureSensorERR  DataStoreElements=PressureSensorERR  IndexOptions=Index vector (dialog)  Indices=1  OutputSizes=1
  Data Store Write15 : DataStoreWrite  DataStoreName=PressureSensorNoCal  DataStoreElements=PressureSensorNoCal  IndexOptions=Index vector (dialog)  Indices=1  OutputSizes=1
  Data Store Write16 : DataStoreWrite  DataStoreName=EHBVoltageLow1  DataStoreElements=EHBVoltageLow1  IndexOptions=Index vector (dialog)  Indices=1  OutputSizes=1
  Data Store Write17 : DataStoreWrite  DataStoreName=EHBVoltageLow2  IndexOptions=Index vector (dialog)  Indices=1  OutputSizes=1
  Data Store Write18 : DataStoreWrite  DataStoreName=EHBVoltageHigh1  DataStoreElements=EHBVoltageHigh1  IndexOptions=Index vector (dialog)  Indices=1  OutputSizes=1
  Data Store Write19 : DataStoreWrite  DataStoreName=EHBVoltageHigh2  DataStoreElements=EHBVoltageHigh2  IndexOptions=Index vector (dialog)  Indices=1  OutputSizes=1
  Data Store Write2 : DataStoreWrite  DataStoreName=CurrentSensorUOverride  IndexOptions=Index vector (dialog)  Indices=1  OutputSizes=1
  Data Store Write20 : DataStoreWrite  DataStoreName=KL15VoltageLow  DataStoreElements=KL15VoltageLow  IndexOptions=Index vector (dialog)  Indices=1  OutputSizes=1
  Data Store Write21 : DataStoreWrite  DataStoreName=KL15VoltageHigh  DataStoreElements=KL15VoltageHigh  IndexOptions=Index vector (dialog)  Indices=1  OutputSizes=1
  Data Store Write22 : DataStoreWrite  DataStoreName=Mot_locked_err  IndexOptions=Index vector (dialog)  Indices=1  OutputSizes=1
  Data Store Write3 : DataStoreWrite  DataStoreName=CurrentSensorVOverride  IndexOptions=Index vector (dialog)  Indices=1  OutputSizes=1
  Data Store Write4 : DataStoreWrite  DataStoreName=CurrentSensorWOverride  IndexOptions=Index vector (dialog)  Indices=1  OutputSizes=1
  Data Store Write5 : DataStoreWrite  DataStoreName=TempSensorOverride  IndexOptions=Index vector (dialog)  Indices=1  OutputSizes=1
  Data Store Write6 : DataStoreWrite  DataStoreName=Err5v  IndexOptions=Index vector (dialog)  Indices=1  OutputSizes=1
  Data Store Write7 : DataStoreWrite  DataStoreName=Chip7189_err  IndexOptions=Index vector (dialog)  Indices=1  OutputSizes=1
  Data Store Write8 : DataStoreWrite  DataStoreName=SpeedSensorOverride  IndexOptions=Index vector (dialog)  Indices=1  OutputSizes=1
  Data Store Write9 : DataStoreWrite  DataStoreName=AngleSensorSignalOverride  DataStoreElements=AngleSensorSignalOverride  IndexOptions=Index vector (dialog)  Indices=1  OutputSizes=1
  Data Type Conversion{1..23} (23 alike) : DataTypeConversion  SaturateOnIntegerOverflow=off  RndMeth=Floor
  wires:
  Data Type Conversion14/1 -> Data Store Write14/1
  Data Type Conversion18/1 -> Data Store Write18/1
  Data Type Conversion15/1 -> Data Store Write15/1
  Data Type Conversion16/1 -> Data Store Write16/1
  Data Type Conversion21/1 -> Data Store Write21/1
  Data Type Conversion17/1 -> Data Store Write17/1
  Data Type Conversion19/1 -> Data Store Write19/1
  Data Type Conversion12/1 -> Data Store Write12/1
  Data Type Conversion9/1 -> Data Store Write9/1
  Data Type Conversion10/1 -> Data Store Write10/1
  DIAG_BUS/1 -> Bus Selector4/1
  Data Type Conversion20/1 -> Data Store Write20/1
  Data Type Conversion11/1 -> Data Store Write11/1
  Data Type Conversion13/1 -> Data Store Write13/1
  Bus Selector4/1 -> Data Type Conversion9/1  "<AngleSensorSignalOverride>"
  Bus Selector4/2 -> Data Type Conversion10/1  "<AngleSensorSignalLost>"
  Bus Selector4/3 -> Data Type Conversion11/1  "<AngleSensorNoCal>"
  Bus Selector4/4 -> Data Type Conversion12/1  "<PressureFlowERR1>"
  Bus Selector4/5 -> Data Type Conversion13/1  "<PressureFlowERR2>"
  Bus Selector4/6 -> Data Type Conversion14/1  "<PressureSensorERR>"
  Bus Selector4/7 -> Data Type Conversion15/1  "<PressureSensorNoCal>"
  Bus Selector4/8 -> Data Type Conversion16/1  "<EHBVoltageLow1>"
  Bus Selector4/9 -> Data Type Conversion17/1  "<EHBVoltageLow2>"
  Bus Selector4/10 -> Data Type Conversion18/1  "<EHBVoltageHigh1>"
  Bus Selector4/11 -> Data Type Conversion19/1  "<EHBVoltageHigh2>"
  Data Type Conversion1/1 -> Data Store Write/1
  Data Type Conversion2/1 -> Data Store Write1/1
  Bus Selector4/12 -> Data Type Conversion1/1  "<LogicVoltageLow>"
  Bus Selector4/13 -> Data Type Conversion2/1  "<LogicVoltageHigh>"
  Bus Selector4/14 -> Data Type Conversion20/1  "<KL15VoltageLow>"
  Bus Selector4/15 -> Data Type Conversion21/1  "<KL15VoltageHigh>"
  Bus Selector4/16 -> Data Type Conversion4/1  "<CurrentSensorUOverride>"
  Bus Selector4/17 -> Data Type Conversion5/1  "<CurrentSensorVOverride>"
  Bus Selector4/18 -> Data Type Conversion6/1  "<CurrentSensorWOverride>"
  Bus Selector4/19 -> Data Type Conversion7/1  "<TempSensorOverride>"
  Bus Selector4/20 -> Data Type Conversion3/1  "<5vErr>"
  Bus Selector4/21 -> Data Type Conversion8/1  "<Chip7189_err>"
  Bus Selector4/22 -> Data Type Conversion22/1  "<SpeedSensorOverride>"
  Bus Selector4/23 -> Data Type Conversion23/1  "<Mot_locked_err>"
  Data Type Conversion4/1 -> Data Store Write2/1
  Data Type Conversion5/1 -> Data Store Write3/1
  Data Type Conversion6/1 -> Data Store Write4/1
  Data Type Conversion7/1 -> Data Store Write5/1
  Data Type Conversion8/1 -> Data Store Write7/1
  Data Type Conversion3/1 -> Data Store Write6/1
  Data Type Conversion22/1 -> Data Store Write8/1
  Data Type Conversion23/1 -> Data Store Write22/1

== system EHB_MOTOR/EHB_MOTOR_PRO/DIAG/EHBDiag ==
  note: EHB电源电压过高
  note: 200ms
  note: EHB电源电压过低
  EHBVoltage : Inport
  Chart : Stateflow chart  TreatAsAtomicUnit=on
  Subsystem : Subsystem
  EHBVoltageLow1 : Outport  VectorParamsAs1DForOutWhenUnconnected=off
  EHBVoltageLow2 : Outport  Port=2  VectorParamsAs1DForOutWhenUnconnected=off
  EHBVoltageHigh1 : Outport  Port=3  VectorParamsAs1DForOutWhenUnconnected=off
  EHBVoltageHigh2 : Outport  Port=4  VectorParamsAs1DForOutWhenUnconnected=off
  wires:
  EHBVoltage/1 -> Subsystem/1(In1)
  Subsystem/1(EHBVoltageLow1) -> EHBVoltageLow1/1
  Chart/1(task_200ms()) -> Subsystem/Trigger
  Subsystem/3(EHBVoltageHigh1) -> EHBVoltageHigh1/1
  Subsystem/2(EHBVoltageLow2) -> EHBVoltageLow2/1
  Subsystem/4(EHBVoltageHigh2) -> EHBVoltageHigh2/1

== system EHB_MOTOR/EHB_MOTOR_PRO/DIAG/KL15VoltageDiag ==
  note: KL15电压过低
  note: 200ms
  note: KL15电压过高
  KL15Voltage : Inport
  Chart : Stateflow chart  TreatAsAtomicUnit=on
  Subsystem : Subsystem
  KL15VoltageLow : Outport  VectorParamsAs1DForOutWhenUnconnected=off
  KL15VoltageHigh : Outport  Port=2  VectorParamsAs1DForOutWhenUnconnected=off
  wires:
  Subsystem/2(KL15VoltageHigh) -> KL15VoltageHigh/1
  Chart/1(task_200ms()) -> Subsystem/Trigger
  Subsystem/1(KL15VoltageLow) -> KL15VoltageLow/1
  KL15Voltage/1 -> Subsystem/1(KL15Voltage)

== system EHB_MOTOR/EHB_MOTOR_PRO/DIAG/LogicVoltageDiag ==
  note: 12VLogic电源电压过高
  note: 200ms
  note: 12VLogic电源电压过低
  LogicVoltage : Inport
  Chart : Stateflow chart  TreatAsAtomicUnit=on
  Subsystem : Subsystem
  LogicVoltageLow : Outport  VectorParamsAs1DForOutWhenUnconnected=off
  LogicVoltageHigh : Outport  Port=2  VectorParamsAs1DForOutWhenUnconnected=off
  wires:
  LogicVoltage/1 -> Subsystem/1(In1)
  Subsystem/1(Out1) -> LogicVoltageLow/1
  Chart/1(task_200ms()) -> Subsystem/Trigger
  Subsystem/2(Out2) -> LogicVoltageHigh/1

== system EHB_MOTOR/EHB_MOTOR_PRO/DIAG/MotLockDiag ==
  In1 : Inport
  Abs : Abs  SaturateOnIntegerOverflow=off
  Abs1 : Abs  SaturateOnIntegerOverflow=off
  Abs2 : Abs  SaturateOnIntegerOverflow=off
  Bus Selector : BusSelector  OutputSignals=Feedback.TEMP_DELAY.EHB_Mot_length,AI_BUS.EHB_iU_filtered,AI_BUS.EHB_iV_filtered,AI_BUS.EHB_iW_filtered
  Constant : Constant  Value=2
  Constant1 : Constant  Value=70
  Constant2 : Constant  Value=70
  Constant3 : Constant  Value=70
  Constant4 : Constant  Value=0  OutDataTypeStr=uint8
  Data Store Memory1 : DataStoreMemory  DataStoreName=tiMotLocked_C  ReadBeforeWriteMsg=warning  WriteAfterWriteMsg=warning  WriteAfterReadMsg=warning  ShowAdditionalParam=off  OutDataTypeStr=uint16
  Data Store Read : DataStoreRead  DataStoreName=tiMotLocked_C  DataStoreElements=tiMotLocked_C  IndexOptions=Index vector (dialog)  Indices=1  OutputSizes=1
  ErrorSignalCount : Stateflow chart  TreatAsAtomicUnit=on
  Logical Operator : Logic  Operator=OR  Inputs=3  AllPortsSameDT=off  OutDataTypeStr=boolean
  Logical Operator1 : Logic  AllPortsSameDT=off  OutDataTypeStr=boolean
  Relational Operator : RelationalOperator  Operator=<  OutDataTypeStr=boolean  RndMeth=Simplest  InputSameDT=off
  Relational Operator1 : RelationalOperator  Operator=>  OutDataTypeStr=boolean  RndMeth=Simplest  InputSameDT=off
  Relational Operator2 : RelationalOperator  Operator=>  OutDataTypeStr=boolean  RndMeth=Simplest  InputSameDT=off
  Relational Operator3 : RelationalOperator  Operator=>  OutDataTypeStr=boolean  RndMeth=Simplest  InputSameDT=off
  Mot_locked_err : Outport  VectorParamsAs1DForOutWhenUnconnected=off
  wires:
  In1/1 -> Bus Selector/1
  Bus Selector/1 -> Relational Operator/1  "<EHB_Mot_length>"
  Constant/1 -> Relational Operator/2
  Constant1/1 -> Relational Operator1/2
  Bus Selector/2 -> Abs/1  "<EHB_iU_filtered>"
  Constant2/1 -> Relational Operator2/2
  Constant3/1 -> Relational Operator3/2
  Bus Selector/4 -> Abs2/1  "<EHB_iW_filtered>"
  Bus Selector/3 -> Abs1/1  "<EHB_iV_filtered>"
  Relational Operator1/1 -> Logical Operator/1
  Relational Operator2/1 -> Logical Operator/2
  Relational Operator3/1 -> Logical Operator/3
  Logical Operator/1 -> Logical Operator1/2
  Relational Operator/1 -> Logical Operator1/1
  Logical Operator1/1 -> ErrorSignalCount/1(Mot_locked)
  Abs/1 -> Relational Operator1/1
  Abs1/1 -> Relational Operator2/1
  Abs2/1 -> Relational Operator3/1
  Constant4/1 -> ErrorSignalCount/3(Recover)
  ErrorSignalCount/1(Mot_locked_err) -> Mot_locked_err/1
  Data Store Read/1 -> ErrorSignalCount/2(tiMotLocked_C)

== system EHB_MOTOR/EHB_MOTOR_PRO/DIAG/MotorDiag ==
  note: 200ms
  note: 电机回路故障
  note: 200ms
  note: 电机过温
  note: 电机过流故障
  note: 200ms
  MotorCircuitCurrent : Inport
  Motor_PWMout : Inport  Port=2
  MotorTemp : Inport  Port=3
  MotorCurrent : Inport  Port=4
  Chart : Stateflow chart  TreatAsAtomicUnit=on
  Chart1 : Stateflow chart  TreatAsAtomicUnit=on
  Chart2 : Stateflow chart  TreatAsAtomicUnit=on
  Subsystem : Subsystem
  Subsystem1 : Subsystem
  Subsystem2 : Subsystem
  MotorCircuitCurrentOverride : Outport  VectorParamsAs1DForOutWhenUnconnected=off
  MotorTempOverride : Outport  Port=2  VectorParamsAs1DForOutWhenUnconnected=off
  MotorCurrentOverride : Outport  Port=3  VectorParamsAs1DForOutWhenUnconnected=off
  wires:
  Subsystem1/1(Out1) -> MotorTempOverride/1
  Chart1/1(task_200ms()) -> Subsystem1/Trigger
  Chart/1(task_200ms()) -> Subsystem/Trigger
  Subsystem/1(Out1) -> MotorCircuitCurrentOverride/1
  MotorCircuitCurrent/1 -> Subsystem/1(In1)
  MotorTemp/1 -> Subsystem1/1(In1)
  MotorCurrent/1 -> Subsystem2/1(In1)
  Subsystem2/1(Out1) -> MotorCurrentOverride/1
  Chart2/1(task_200ms()) -> Subsystem2/Trigger
  Motor_PWMout/1 -> Subsystem/2(Motor_PWMout)

== system EHB_MOTOR/EHB_MOTOR_PRO/DIAG/PWMCircuitDiag ==
  note: PWM波发送电路故障
  In1 : Inport
  Ground : Ground
  Terminator : Terminator
  PWMCircuitErr : Outport  VectorParamsAs1DForOutWhenUnconnected=off
  wires:
  In1/1 -> Terminator/1
  Ground/1 -> PWMCircuitErr/1

== system EHB_MOTOR/EHB_MOTOR_PRO/DIAG/PressureSensorDiag ==
  note: 200ms
  note: 200ms
  note: 压力跟随故障
  note: 200ms
  note: 压力传感器故障
  note: 压力传感器缺少标定
  VCU_Brake_AimPressure : Inport
  EHB_actPresure_filtered : Inport  Port=2
  EHB_Presure_ADC : Inport  Port=3
  PressureSensorCalFlag : Inport  Port=4
  Chart : Stateflow chart  TreatAsAtomicUnit=on
  Chart1 : Stateflow chart  TreatAsAtomicUnit=on
  Chart2 : Stateflow chart  TreatAsAtomicUnit=on
  Subsystem : Subsystem
  Subsystem1 : Subsystem
  Subsystem2 : Subsystem
  PressureFlowERR1 : Outport  VectorParamsAs1DForOutWhenUnconnected=off
  PressureFlowERR2 : Outport  Port=2  VectorParamsAs1DForOutWhenUnconnected=off
  PressureSensorERR : Outport  Port=3  VectorParamsAs1DForOutWhenUnconnected=off
  PressureSensorNoCal : Outport  Port=4  VectorParamsAs1DForOutWhenUnconnected=off
  wires:
  Chart2/1(task_200ms()) -> Subsystem2/Trigger
  Subsystem2/1(Out1) -> PressureSensorNoCal/1
  EHB_actPresure_filtered/1 -> Subsystem/2(EHB_actPresure_filtered)
  Subsystem1/1(Out1) -> PressureSensorERR/1
  Chart1/1(task_200ms()) -> Subsystem1/Trigger
  Chart/1(task_200ms()) -> Subsystem/Trigger
  Subsystem/1(Out1) -> PressureFlowERR1/1
  PressureSensorCalFlag/1 -> Subsystem2/1(In1)
  VCU_Brake_AimPressure/1 -> Subsystem/1(VCU_Brake_AimPressure)
  Subsystem/2(Out2) -> PressureFlowERR2/1
  EHB_Presure_ADC/1 -> Subsystem1/1(EHB_Presure_ADC)

== system EHB_MOTOR/EHB_MOTOR_PRO/DIAG/RespondOvertimeDiag ==
  note: 响应超时故障
  In1 : Inport
  Ground : Ground
  Terminator : Terminator
  Chip7189_err : Outport  VectorParamsAs1DForOutWhenUnconnected=off
  wires:
  Ground/1 -> Chip7189_err/1
  In1/1 -> Terminator/1

== system EHB_MOTOR/EHB_MOTOR_PRO/DIAG/SpeedSensorDiag ==
  note: 200ms
  note: 轮速传感器信号电压异常
  SpeedSensor : Inport
  Chart : Stateflow chart  TreatAsAtomicUnit=on
  Subsystem : Subsystem
  SpeedSensorOverride : Outport  VectorParamsAs1DForOutWhenUnconnected=off
  wires:
  SpeedSensor/1 -> Subsystem/1(In1)
  Chart/1(task_200ms()) -> Subsystem/Trigger
  Subsystem/1(Out1) -> SpeedSensorOverride/1
